simulink model "convert_cel_to"  (R2021a)
settings: Solver=VariableStepAuto  StartTime=0.0  StopTime=10.0  RelTol=1e-3
values from neighbouring files (symbols this model uses):
  X = input(prompt)    [project_2.m]
settings Model: Creator=rmudi  LastModifiedBy=rmudi

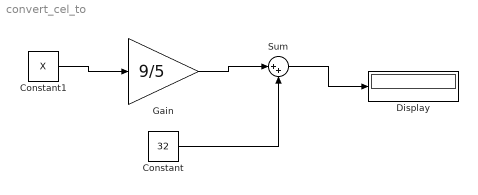
== system convert_cel_to ==
  Constant : Constant  Value=32
  Constant1 : Constant  Value=X
  Display : Display
  Gain : Gain  Gain=9/5
  Sum : Sum  Inputs=|++
  wires:
  Gain/1 -> Sum/1
  Constant/1 -> Sum/2
  Constant1/1 -> Gain/1
  Sum/1 -> Display/1
